simulink model "TestingModels"  (R2021b)
settings: Solver=VariableStepAuto  StartTime=0.0  StopTime=120  FixedStep=1  RelTol=1e-3
settings Model: Creator=mariodelossantos  LastModifiedBy=mariodelossantos

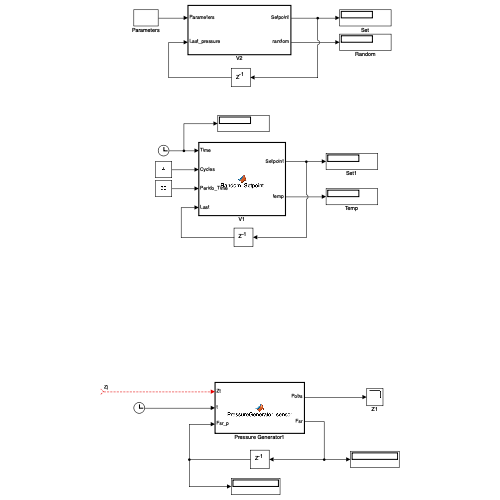
[thumbnail: Simulink's stored preview of the top-level diagram]
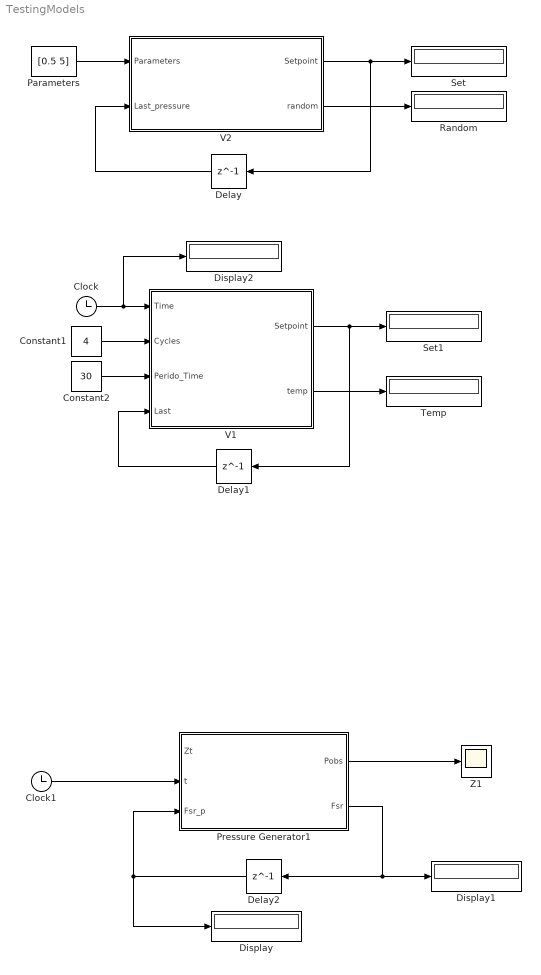
== system TestingModels ==
  Clock : Clock
  Clock1 : Clock
  Constant1 : Constant  Value=4
  Constant2 : Constant  Value=30
  Delay : Delay  DelayLength=1  InitialCondition=0
  Delay1 : Delay  DelayLength=1  InitialCondition=0
  Delay2 : Delay  DelayLength=1  InitialCondition=0.0001
  Display : Display
  Display1 : Display
  Display2 : Display
  Parameters : Constant  Value=[0.5 5]
  Pressure Generator1 : MATLAB Function  TreatAsAtomicUnit=on
  Random : Display
  Set : Display
  Set1 : Display
  Temp : Display
  V1 : MATLAB Function  TreatAsAtomicUnit=on
  V2 : MATLAB Function  TreatAsAtomicUnit=on
  Z1 : Scope
  wires:
  Delay/1 -> V2/2(Last_pressure)
  Parameters/1 -> V2/1(Parameters)
  V2/1(Setpoint) -> Delay/1, Set/1
  V2/2(random) -> Random/1
  V1/1(Setpoint) -> Delay1/1, Set1/1
  Delay1/1 -> V1/4(Last)
  Constant1/1 -> V1/2(Cycles)
  Clock/1 -> Display2/1, V1/1(Time)
  Constant2/1 -> V1/3(Perido_Time)
  V1/2(temp) -> Temp/1
  ? -> Pressure Generator1/1(Zt)  "Zj"
  Delay2/1 -> Display/1, Pressure Generator1/3(Fsr_p)
  Clock1/1 -> Pressure Generator1/2(t)
  Pressure Generator1/2(Fsr) -> Delay2/1, Display1/1
  Pressure Generator1/1(Pobs) -> Z1/1

== matlab function TestingModels/V1 ==
  settings: updateMethod=DISCRETE
  data: Setpoint output; Time input; Cycles input; Perido_Time input; Last input; temp output
function [Setpoint, temp] = Random_Setpoint(Time, Cycles,Perido_Time, Last)
    Pcycles = ones(Cycles);
    temp = 0;
    min = 0;
    max = 8;
    r = min + rand(1)*(max-min);
    for i = 1:Cycles
        Pcycles(i) = i;
        Pcycles(i) = i*Perido_Time;
        %We should fine a random criteria to change the setpoint, not just
        %time, or the moment B changes. For now works to demostrate the
        %control without fNIRS
         if (Time > (Pcycles(i)-0.5)) && (Time < (Pcycles(i)+1))
            %disp("Time")
            %disp(Time)
            temp = r;
            %disp("Setpoint")
            %disp(temp)
        else 
            temp = Last;
        end  
    end

    Setpoint = temp;

== matlab function TestingModels/V2 ==
  settings: updateMethod=DISCRETE
  data: Setpoint output; Parameters input; Last_pressure input; random output
function [Setpoint, random] = Random_Setpoint(Parameters, Last_pressure)


    %Parameters = [threshold Start_setpoint]

    %Random used to simulate the connectivity changes, so we must change
    %the pressure setpoint when changes in the connectitvy are observed.
    tmin = 0;
    tmax = 5;
        %We should fine a random criteria to change the setpoint, not just
        %time, or the moment B changes. For now works to demostrate the
        %control without fNIRS
    random = tmin + rand(1) * (tmax - tmin);

    temp = 0;
   %Pressure Setpoint selection
    pmin = 0;
    pmax = 8;
    new_pressure = pmin + rand(1)*(pmax-pmin);
         if (random < Parameters(1))
            %disp("Time")
            %disp(Time)
            temp = new_pressure;
            %disp("Setpoint")
            %disp(temp)
        else 
            temp = Last_pressure;
                if (Parameters(2) == temp || temp == 0)
                    temp = Parameters(2);
                else
                    temp = Last_pressure;
                end
        end  

    Setpoint = temp;

== matlab function TestingModels/Pressure Generator1 ==
  data: Zt input; Pobs output; t input; Fsr_p input; Fsr output
function [Pobs,Fsr] = PressureGenerator_sensor(Zt, t,Fsr_p)
    C = 0.000001; % 0.1uF
    Vcc = 500; %Considering 5V as a real sensor, the value is on mV
    Rf = 10000; %Fixed resistor 10k ohms
    kgf = 0.1019716213; % 1N = 0.1019716213 kgf
    Fsr = 0;
    Fsrforce = 0;

    Vout = Zt(1) * (1 - exp( -t / C)); %Emulation of the capacitor
    Fsr = (Vcc - Vout * Rf) / Vout;
    FsConductance = 1000000; %Sensor conductance in uOhms
    FsConductance = FsConductance / Fsr;
    if FsConductance <= 1000
        Fsrforce = FsConductance / 80; %Force on Newtons
    else
        Fsrforce = FsConductance - 1000;
        Fsrforce = Fsrforce / 30;
    end
    
Pobs = Fsrforce* kgf;

end
